simulink model "bandwidth_force_sea"  (R2020b)
settings: Solver=ode4  StartTime=0.0  StopTime=5  FixedStep=1e-5  MaxStep=1e-4  RelTol=1e-4  EnableMultiTasking=on
values from neighbouring files (symbols this model uses):
  D = 0.9    [siciliano_position_params.m]
  dm = 0.0068    [siciliano_position_params.m]
  FF = 0    [siciliano_position_params.m]
  Jm = 0.0104    [siciliano_position_params.m]
  P = 10    [siciliano_position_params.m]
undefined symbols (not defined in the file or in its folder): Be, Bl, Je, Jl, Ke, Ks, qe
settings Model: Creator=eldisondimo  LastModifiedBy=filippo
settings DataIOCC: LimitDataPoints=on  SaveOutput=off  SaveTime=off  ReturnWorkspaceOutputs=off
settings OptimizationCC: ExpressionDepthLimit=2147483647  LifeSpan=1
settings DebuggingCC: UnderspecifiedInitializationDetection=Classic  MergeDetectMultiDrivingBlocksExec=none  FcnCallInpInsideContextMsg=warning  AllowSymbolicDim=off  StateNameClashWarn=warning  SFUnexpectedBacktrackingDiag=warning  SFNoUnconditionalDefaultTransitionDiag=warning  SFExecutionAtInitializationDiag=none  ArithmeticOperatorsInVariantConditions=warning
settings SFSimCC: SimUseLocalCustomCode=off  CustomCodeUndefinedFunction=UseInterfaceOnly
settings RTWCC: RTWUseLocalCustomCode=off
settings CodeAppCC: StateflowObjectComments=on
settings GRTTargetCC: TargetLangStandard=C89/C90 (ANSI)  CombineOutputUpdateFcns=off  GRTInterface=on

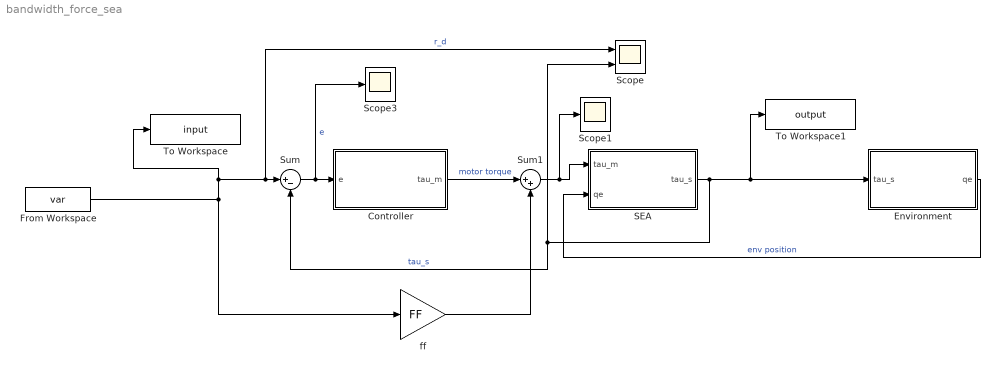
== system bandwidth_force_sea ==
  Controller : Subsystem
  Environment : Subsystem
  From Workspace : FromWorkspace  VariableName=var
  SEA : Subsystem
  Scope : Scope  NumInputPorts=2
  Scope1 : Scope
  Scope3 : Scope
  Sum : Sum  Inputs=|+-
  Sum1 : Sum  Inputs=|++
  To Workspace : ToWorkspace  VariableName=input  SaveFormat=Structure With Time  SampleTime=-1
  To Workspace1 : ToWorkspace  VariableName=output  SaveFormat=Structure With Time  SampleTime=-1
  "ff " : Gain  Gain=FF
  wires:
  Sum/1 -> Scope3/1, Controller/1(e)  "e"
  SEA/1(tau_s) -> Scope/2, Sum/2, To Workspace1/1, Environment/1(tau_s)  "tau_s"
  Controller/1(tau_m) -> Sum1/1  "motor torque"
  Environment/1(qe) -> SEA/2("qe ")  "env position"
  "ff "/1 -> Sum1/2
  From Workspace/1 -> "ff "/1, To Workspace/1, Scope/1, Sum/1  "r_d"
  Sum1/1 -> Scope1/1, SEA/1(tau_m)

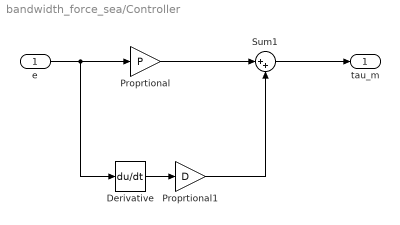
== system bandwidth_force_sea/Controller ==
  e : Inport
  Derivative : Derivative
  Proprtional : Gain  Gain=P
  Proprtional1 : Gain  Gain=D
  Sum1 : Sum  Inputs=|++
  tau_m : Outport  VectorParamsAs1DForOutWhenUnconnected=off
  wires:
  e/1 -> Derivative/1, Proprtional/1
  Sum1/1 -> tau_m/1
  Derivative/1 -> Proprtional1/1
  Proprtional/1 -> Sum1/1
  Proprtional1/1 -> Sum1/2

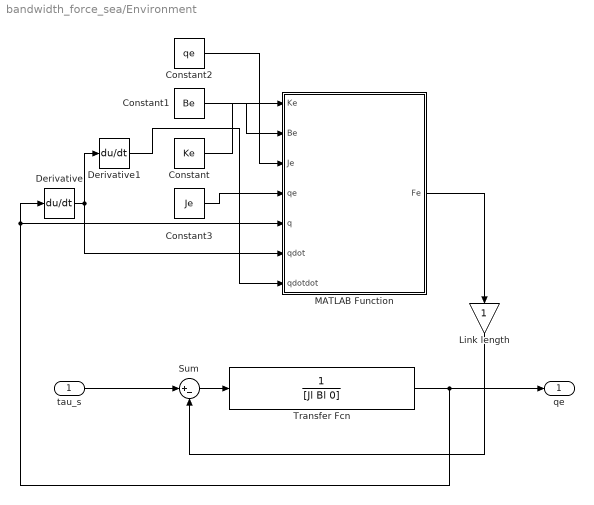
== system bandwidth_force_sea/Environment ==
  tau_s : Inport
  Constant : Constant  Value=Ke
  Constant1 : Constant  Value=Be
  Constant2 : Constant  Value=qe
  Constant3 : Constant  Value=Je
  Derivative : Derivative
  Derivative1 : Derivative
  Link length : Gain
  MATLAB Function : MATLAB Function  TreatAsAtomicUnit=on
  Sum : Sum  Inputs=|+-
  Transfer Fcn : TransferFcn  Denominator=[Jl Bl 0]
  qe : Outport  VectorParamsAs1DForOutWhenUnconnected=off
  wires:
  tau_s/1 -> Sum/1
  Derivative/1 -> Derivative1/1, MATLAB Function/6(qdot)
  MATLAB Function/1(Fe) -> Link length/1
  Sum/1 -> Transfer Fcn/1
  Transfer Fcn/1 -> Derivative/1, MATLAB Function/5(q), qe/1
  Constant/1 -> MATLAB Function/1(Ke)
  Constant1/1 -> MATLAB Function/2(Be)
  Link length/1 -> Sum/2
  Derivative1/1 -> MATLAB Function/7(qdotdot)
  Constant3/1 -> MATLAB Function/4(qe)
  Constant2/1 -> MATLAB Function/3(Je)

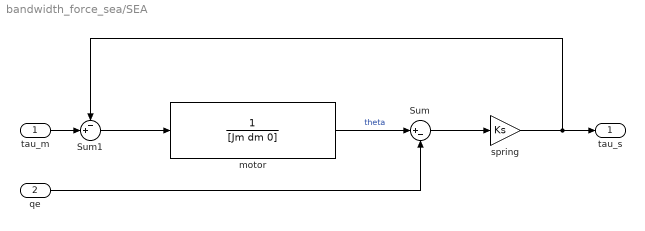
== system bandwidth_force_sea/SEA ==
  tau_m : Inport
  "qe " : Inport  Port=2
  Sum : Sum  Inputs=|+-
  Sum1 : Sum  Inputs=-+|
  "motor " : TransferFcn  Denominator=[Jm dm 0]
  "spring " : Gain  Gain=Ks
  tau_s : Outport  VectorParamsAs1DForOutWhenUnconnected=off
  wires:
  "motor "/1 -> Sum/1  "theta"
  "qe "/1 -> Sum/2
  Sum/1 -> "spring "/1
  "spring "/1 -> Sum1/1, tau_s/1
  tau_m/1 -> Sum1/2
  Sum1/1 -> "motor "/1

== matlab function bandwidth_force_sea/Environment/MATLAB Function ==
  data: Ke input; Be input; Je input; qe input; Fe output; q input; qdot input; qdotdot input
function Fe = envModel(Ke, Be, Je, qe, q, qdot, qdotdot)

% if q > qe
    Fe = Ke * (q - qe) + Be * qdot + Je * qdotdot;
% else
%     Fe = 0;
end
